simulink model "Simulation"  (R2016a)
settings: Solver=VariableStepAuto  StartTime=0.0  StopTime=5  FixedStep=1e-6  RelTol=1e-3
values from neighbouring files (symbols this model uses):
  B = 0    [Main.m]
  di_k_init = rand(2, 8)    [Main.m]
  G = (1/3)*[2 -1 -1; 0 sqrt(3) -sqrt(3)]    [Main.m]
  i_cmd_init = zeros(2, 3)    [Main.m]
  i_future_init = rand(2, 8)    [Main.m]
  i_k_init = rand(2, 8)    [Main.m]
  I_output = zeros(3, 1)    [Main.m]
  i_prev_init = rand(2, 1)    [Main.m]
  J = 0.0755    [Main.m]
  Ld = 0.04    [Main.m]
  Lq = 0.016    [Main.m]
  P = 3    [Main.m]
  R = 2.5    [Main.m]
  r_init = [0; 50; 0]    [Main.m]
  S_init = ones(3, 1)    [Main.m]
  Sensor_output = zeros(2, 1)    [Main.m]
  Ts = 100e-6    (= 0.0001)    [Main.m]
  V = 220    [Main.m]
libraries: simulink x1
settings Model: Creator=Raheel  LastModifiedBy=Raheel

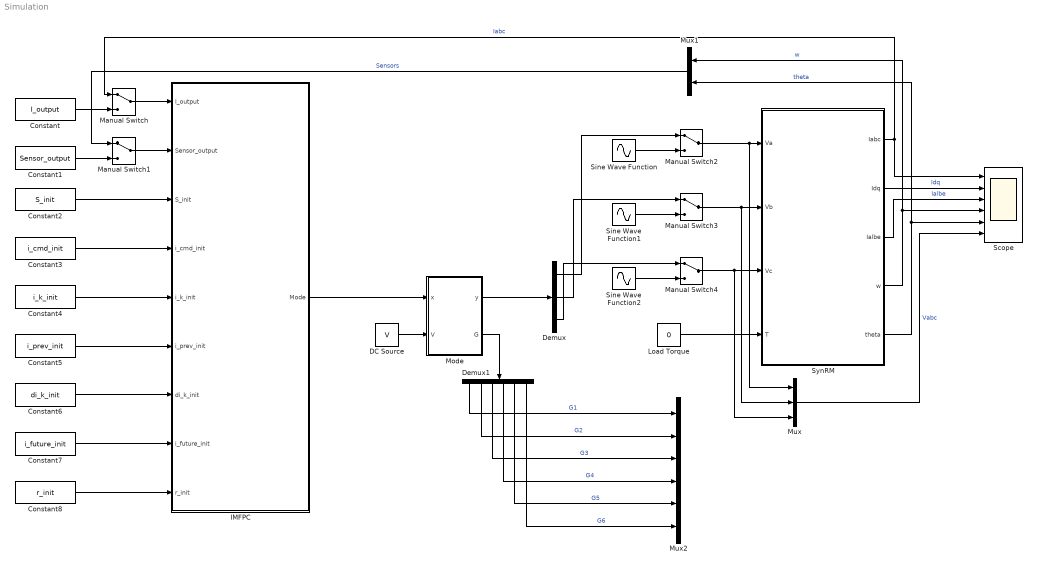
== system Simulation ==
  Constant : Constant  Value=I_output  VectorParams1D=off  SampleTime=Ts
  Constant1 : Constant  Value=Sensor_output  VectorParams1D=off  SampleTime=Ts
  Constant2 : Constant  Value=S_init  VectorParams1D=off  SampleTime=Ts
  Constant3 : Constant  Value=i_cmd_init  VectorParams1D=off  SampleTime=Ts
  Constant4 : Constant  Value=i_k_init  VectorParams1D=off  SampleTime=Ts
  Constant5 : Constant  Value=i_prev_init  SampleTime=Ts
  Constant6 : Constant  Value=di_k_init  SampleTime=Ts
  Constant7 : Constant  Value=i_future_init  SampleTime=Ts
  Constant8 : Constant  Value=r_init  SampleTime=Ts
  DC Source : Constant  Value=V  SampleTime=Ts
  Demux : Demux  Outputs=3
  Demux1 : Demux  Outputs=6
  IMFPC : Subsystem
  "Load Torque " : Constant  Value=0  SampleTime=0
  Manual Switch{,1..4} (5 alike) : ManualSwitch
  Mode : MATLAB Function  TreatAsAtomicUnit=on
  Mux : Mux  Inputs=3
  Mux1 : Mux  Inputs=2
  Mux2 : Mux  Inputs=6
  Scope : Scope  NumInputPorts=6
  Sine Wave Function : Sin  Amplitude=V  Frequency=50  SampleTime=0
  Sine Wave Function1 : Sin  Amplitude=V  Frequency=50  Phase=-2*pi/3  SampleTime=0
  Sine Wave Function2 : Sin  Amplitude=V  Frequency=50  Phase=2*pi/3  SampleTime=0
  SynRM : Subsystem
  wires:
  Constant8/1 -> IMFPC/9(r_init)
  Constant7/1 -> IMFPC/8(i_future_init)
  Constant6/1 -> IMFPC/7(di_k_init)
  Constant5/1 -> IMFPC/6(i_prev_init)
  Constant4/1 -> IMFPC/5(i_k_init)
  Constant3/1 -> IMFPC/4(i_cmd_init)
  Constant2/1 -> IMFPC/3(S_init)
  "Load Torque "/1 -> SynRM/4(T)
  Sine Wave Function1/1 -> Manual Switch3/2
  Sine Wave Function/1 -> Manual Switch2/2
  Sine Wave Function2/1 -> Manual Switch4/2
  SynRM/1(Iabc) -> Scope/1, Manual Switch/1  "Iabc"
  SynRM/4(w) -> Mux1/1, Scope/4  "w"
  SynRM/5(theta) -> Mux1/2, Scope/5  "theta"
  SynRM/3(Ialbe) -> Scope/3  "Ialbe"
  SynRM/2(Idq) -> Scope/2  "Idq"
  Mux/1 -> Scope/6  "Vabc"
  Constant/1 -> Manual Switch/2
  Manual Switch/1 -> IMFPC/1(I_output)
  Manual Switch1/1 -> IMFPC/2(Sensor_output)
  Constant1/1 -> Manual Switch1/2
  Manual Switch2/1 -> Mux/1, SynRM/1(Va)
  Manual Switch3/1 -> Mux/2, SynRM/2(Vb)
  Manual Switch4/1 -> Mux/3, SynRM/3(Vc)
  IMFPC/1(Mode) -> Mode/1(x)
  DC Source/1 -> Mode/2(V)
  Mode/1(y) -> Demux/1
  Demux/1 -> Manual Switch2/1
  Mux1/1 -> Manual Switch1/1  "Sensors"
  Demux/2 -> Manual Switch3/1
  Demux/3 -> Manual Switch4/1
  Mode/2(G) -> Demux1/1
  Demux1/6 -> Mux2/6  "G6"
  Demux1/5 -> Mux2/5  "G5"
  Demux1/4 -> Mux2/4  "G4"
  Demux1/3 -> Mux2/3  "G3"
  Demux1/2 -> Mux2/2  "G2"
  Demux1/1 -> Mux2/1  "G1"

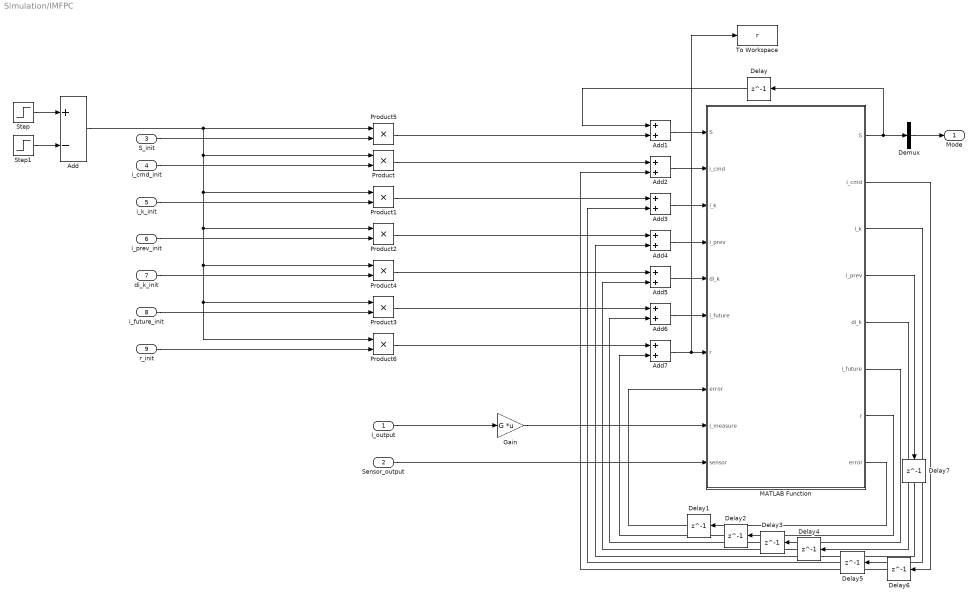
== system Simulation/IMFPC ==
  I_output : Inport
  Sensor_output : Inport  Port=2
  S_init : Inport  Port=3
  i_cmd_init : Inport  Port=4
  i_k_init : Inport  Port=5
  i_prev_init : Inport  Port=6
  di_k_init : Inport  Port=7
  i_future_init : Inport  Port=8
  r_init : Inport  Port=9
  Add : Sum  Inputs=+-
  Add{1..7} (7 alike) : Sum
  Delay{,1..7} (8 alike) : Delay  DelayLength=1  InitialCondition=0  SampleTime=Ts
  Demux : Demux  Outputs=3
  Gain : Gain  Gain=G  Multiplication=Matrix(K*u)
  MATLAB Function : MATLAB Function  TreatAsAtomicUnit=on
  Product{,1..6} (7 alike) : Product
  Step : Step  Time=0  SampleTime=Ts  ZeroCross=off
  Step1 : Step  Time=Ts  SampleTime=Ts  ZeroCross=off
  To Workspace : ToWorkspace  VariableName=r  SaveFormat=Timeseries  SampleTime=-1
  Mode : Outport
  wires:
  Step/1 -> Add/1
  Step1/1 -> Add/2
  MATLAB Function/8(error) -> Delay1/1
  MATLAB Function/1(S) -> Delay/1, Demux/1
  Add/1 -> Product1/1, Product6/1, Product3/1, Product4/1, Product2/1, Product/1, Product5/1
  Product5/1 -> Add1/2
  Add1/1 -> MATLAB Function/1("S ")
  Add2/1 -> MATLAB Function/2("i_cmd ")
  Add3/1 -> MATLAB Function/3("i_k ")
  Add4/1 -> MATLAB Function/4("i_prev ")
  Add5/1 -> MATLAB Function/5("di_k ")
  Add6/1 -> MATLAB Function/6("i_future ")
  Add7/1 -> To Workspace/1, MATLAB Function/7("r ")
  Product/1 -> Add2/1
  Product1/1 -> Add3/1
  Product2/1 -> Add4/1
  Product4/1 -> Add5/1
  Product3/1 -> Add6/1
  Product6/1 -> Add7/1
  MATLAB Function/2(i_cmd) -> Delay6/1
  MATLAB Function/3(i_k) -> Delay5/1
  MATLAB Function/5(di_k) -> Delay4/1
  MATLAB Function/6(i_future) -> Delay3/1
  MATLAB Function/7(r) -> Delay2/1
  Gain/1 -> MATLAB Function/9(i_measure)
  S_init/1 -> Product5/2
  i_cmd_init/1 -> Product/2
  r_init/1 -> Product6/2
  i_future_init/1 -> Product3/2
  di_k_init/1 -> Product4/2
  i_prev_init/1 -> Product2/2
  i_k_init/1 -> Product1/2
  Demux/2 -> Mode/1
  I_output/1 -> Gain/1
  Sensor_output/1 -> MATLAB Function/10(sensor)
  Delay/1 -> Add1/1
  Delay1/1 -> MATLAB Function/8("error ")
  Delay2/1 -> Add7/2
  Delay3/1 -> Add6/2
  Delay4/1 -> Add5/2
  Delay5/1 -> Add3/2
  Delay6/1 -> Add2/2
  MATLAB Function/4(i_prev) -> Delay7/1
  Delay7/1 -> Add4/2

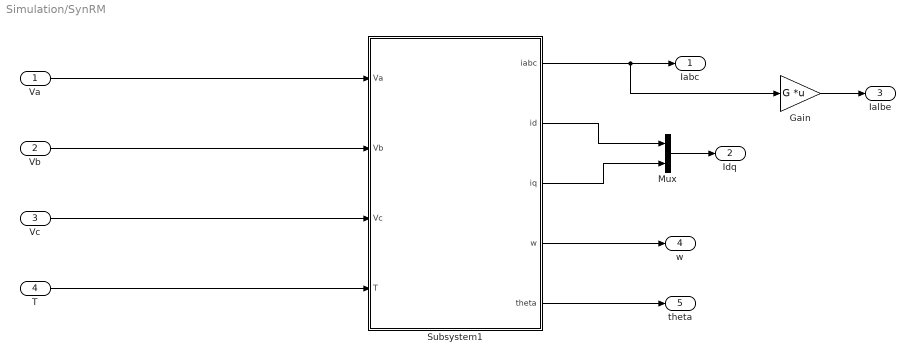
== system Simulation/SynRM ==
  Va : Inport
  Vb : Inport  Port=2
  Vc : Inport  Port=3
  T : Inport  Port=4
  Gain : Gain  Gain=G  Multiplication=Matrix(K*u)
  Mux : Mux  Inputs=2
  Subsystem1 : Subsystem
  Iabc : Outport
  Idq : Outport  Port=2
  Ialbe : Outport  Port=3
  w : Outport  Port=4
  theta : Outport  Port=5
  wires:
  Va/1 -> Subsystem1/1(Va)
  Vb/1 -> Subsystem1/2(Vb)
  Vc/1 -> Subsystem1/3(Vc)
  T/1 -> Subsystem1/4(T)
  Subsystem1/1(iabc) -> Gain/1, Iabc/1
  Subsystem1/2(id) -> Mux/1
  Subsystem1/3(iq) -> Mux/2
  Mux/1 -> Idq/1
  Gain/1 -> Ialbe/1
  Subsystem1/5(theta) -> theta/1
  Subsystem1/4(w) -> w/1

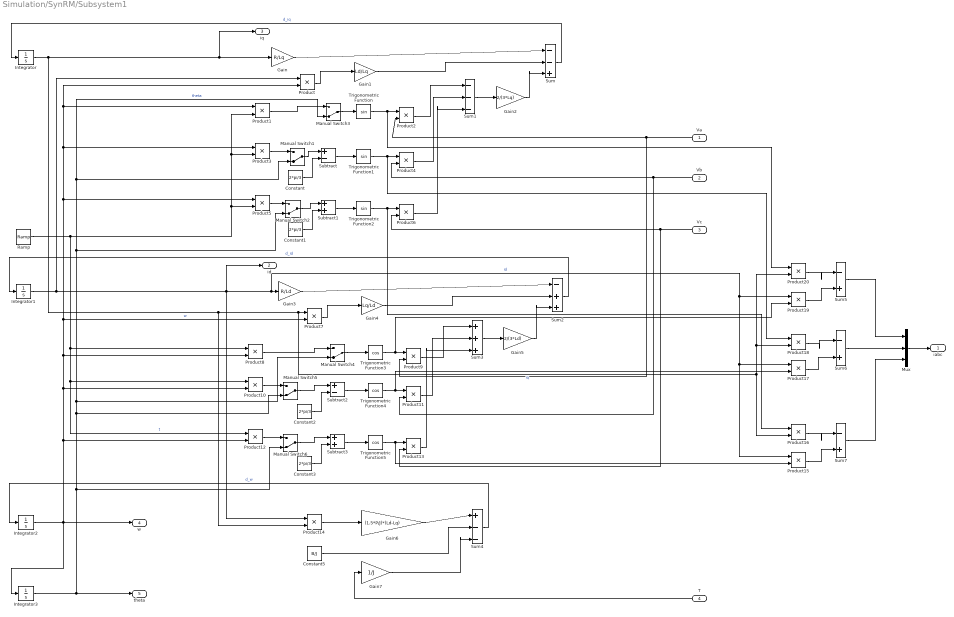
== system Simulation/SynRM/Subsystem1 ==
  Va : Inport
  Vb : Inport  Port=2
  Vc : Inport  Port=3
  T : Inport  Port=4
  Constant{,1..3} (4 alike) : Constant  Value=2*pi/3  SampleTime=0
  Constant5 : Constant  Value=B/J  SampleTime=0
  Gain : Gain  Gain=R/Lq
  Gain1 : Gain  Gain=Ld/Lq
  Gain2 : Gain  Gain=2/(3*Lq)
  Gain3 : Gain  Gain=R/Ld
  Gain4 : Gain  Gain=Lq/Ld
  Gain5 : Gain  Gain=2/(3*Ld)
  Gain6 : Gain  Gain=(1.5*P/J)*(Ld-Lq)
  Gain7 : Gain  Gain=1/J
  Integrator{,1..3} (4 alike) : Integrator
  Manual Switch{1..6} (6 alike) : ManualSwitch  CurrentSetting=0
  Mux : Mux  Inputs=3
  Product{,1..20} (21 alike) : Product
  Ramp : simulink/Sources/Ramp  slope=1  start=0  X0=0
  Subtract : Sum  Inputs=+-
  Subtract1 : Sum
  Subtract2 : Sum  Inputs=+-
  Subtract3 : Sum
  Sum : Sum  Inputs=|--+
  Sum1 : Sum  Inputs=|---
  Sum2 : Sum  Inputs=|-++
  Sum3 : Sum  Inputs=|+++
  Sum4 : Sum  Inputs=|+--
  Sum5 : Sum  Inputs=|-+
  Sum6 : Sum  Inputs=|-+
  Sum7 : Sum  Inputs=|-+
  Trigonometric Function : Trigonometry
  Trigonometric Function1 : Trigonometry
  Trigonometric Function2 : Trigonometry
  Trigonometric Function3 : Trigonometry  Operator=cos
  Trigonometric Function4 : Trigonometry  Operator=cos
  Trigonometric Function5 : Trigonometry  Operator=cos
  iabc : Outport
  id : Outport  Port=2
  iq : Outport  Port=3
  w : Outport  Port=4
  theta : Outport  Port=5
  wires:
  Integrator/1 -> Product14/2, Product16/2, Product20/2, Product18/2, Product7/1, iq/1, Gain/1  "iq"
  Gain/1 -> Sum/1
  Gain1/1 -> Sum/2
  Product/1 -> Gain1/1
  Ramp/1 -> Product8/1, Product10/1, Product12/1, Product1/2, Product3/2, Product5/2  "t"
  Constant/1 -> Subtract/2
  Trigonometric Function1/1 -> Product18/1, Product4/1
  Constant1/1 -> Subtract1/2
  Trigonometric Function2/1 -> Product16/1, Product6/1
  Product2/1 -> Sum1/1
  Product4/1 -> Sum1/2
  Product6/1 -> Sum1/3
  Sum1/1 -> Gain2/1
  Gain2/1 -> Sum/3
  Sum/1 -> Integrator/1  "d_iq"
  Integrator1/1 -> Product14/1, Product19/1, Product17/1, Product15/1, Gain3/1, id/1, Product/1  "id"
  Gain3/1 -> Sum2/1
  Gain4/1 -> Sum2/2
  Product7/1 -> Gain4/1
  Integrator2/1 -> w/1, Integrator3/1, Product10/2, Product8/2, Product7/2, Product5/1, Product3/1, Product1/1, Product/2, Product12/2  "w"
  Trigonometric Function3/1 -> Product19/2, Product9/1
  Va/1 -> Product9/2, Product2/2
  Constant2/1 -> Subtract2/2
  Trigonometric Function4/1 -> Product17/2, Product11/1
  Vb/1 -> Product11/2, Product4/2
  Constant3/1 -> Subtract3/2
  Trigonometric Function5/1 -> Product15/2, Product13/1
  Vc/1 -> Product13/2, Product6/2
  Product9/1 -> Sum3/1
  Product11/1 -> Sum3/2
  Product13/1 -> Sum3/3
  Sum3/1 -> Gain5/1
  Gain5/1 -> Sum2/3
  Sum2/1 -> Integrator1/1  "d_id"
  Product14/1 -> Gain6/1
  Gain6/1 -> Sum4/1
  Sum4/1 -> Integrator2/1  "d_w"
  Constant5/1 -> Sum4/2
  Gain7/1 -> Sum4/3
  T/1 -> Gain7/1
  Integrator3/1 -> Manual Switch6/2, Manual Switch5/2, Manual Switch4/2, Manual Switch2/2, Manual Switch1/2, Manual Switch3/2, theta/1  "theta"
  Trigonometric Function/1 -> Product20/1, Product2/1
  Product20/1 -> Sum5/1
  Product19/1 -> Sum5/2
  Product18/1 -> Sum6/1
  Product17/1 -> Sum6/2
  Product16/1 -> Sum7/1
  Product15/1 -> Sum7/2
  Sum5/1 -> Mux/1
  Mux/1 -> iabc/1
  Sum6/1 -> Mux/2
  Sum7/1 -> Mux/3
  Manual Switch3/1 -> Trigonometric Function/1
  Product1/1 -> Manual Switch3/1
  Manual Switch4/1 -> Trigonometric Function3/1
  Product8/1 -> Manual Switch4/1
  Product3/1 -> Manual Switch1/1
  Manual Switch1/1 -> Subtract/1
  Subtract/1 -> Trigonometric Function1/1
  Product5/1 -> Manual Switch2/1
  Subtract1/1 -> Trigonometric Function2/1
  Manual Switch2/1 -> Subtract1/1
  Product10/1 -> Manual Switch5/1
  Subtract2/1 -> Trigonometric Function4/1
  Manual Switch5/1 -> Subtract2/1
  Product12/1 -> Manual Switch6/1
  Subtract3/1 -> Trigonometric Function5/1
  Manual Switch6/1 -> Subtract3/1

== matlab function Simulation/Mode ==
  data: x input; y output; V input; G output
function [y, G]=Mode(x, V)

switch x
    case 1
        y=[0; 0; 0];
        G=[0; 1; 0; 1; 0; 1];
    case 2
        y=[2*V/3; -V/3; -V/3];
        G=[1; 0; 0; 1; 0; 1];
    case 3
        y=[-2*V/3; V/3; V/3];
        G=[0; 1; 1; 0; 1; 0];
    case 4
        y=[-V/3; 2*V/3; -V/3];
        G=[0; 1; 1; 0; 0; 1];
    case 5
        y=[V/3; -2*V/3; V/3];
        G=[1; 0; 0; 1; 1; 0];
    case 6
        y=[-V/3; -V/3; 2*V/3];
        G=[0; 1; 0; 1; 1; 0];
    case 7
        y=[V/3; V/3; -2*V/3];
        G=[1; 0; 1; 0; 0; 1];
    case 8
        y=[0; 0; 0];
        G=[1; 0; 1; 0; 1; 0];
    otherwise
        disp('Error! Incorrect mode inserted');
        y=[0; 0; 0];
        G=[1; 0; 1; 0; 1; 0];
end

end

== matlab function Simulation/IMFPC/MATLAB Function ==
  data: S input; S output; i_cmd input; i_k input; i_prev input; di_k input; i_future input; r input; error input; i_measure input; sensor input; i_cmd output; i_k output; i_prev output; di_k output; i_future output; r output; error output
%% Details about the algorithm IMPFC
% 1) S is a vector. S(1)=Present mode, S(2)=Mode to be applied, S(3)=Mode calculated
% 2) i_cmd is a matrix. i_cmd(a, 1)=i*(k), i_cmd(a, 2)=i*(k-1), i_cmd(a, 3)=i*(k-2)
%    a=1 means alpha, a=2 means beta.
% 3) i_k is a matrix. i_k(a, b) are the predicted values at present instant.
%    a=1 means alpha, a=2 means beta, b represents the conducting mode.
% 4) i_measure is a vector. i_measure(a) is the current measurement sample.
%    a=1 means alpha, a=2 means beta.
% 5) i_prev is a vector. i_prev(a) is the previous measurement sample.
%    a=1 means alpha, a=2 means beta.
% 6) di_prev is a matrix. di_prev(a, b) is the current variation for previous time instant.
%    a=1 means alpha, a=2 means beta.
% 7) i_future is a matrix. i_future(a, b) are the predicted values at next instant.
%    a=1 means alpha, a=2 means beta, b represents the conducting mode.
% 8) r is a vector. r(1) takes on values from 0 to r(2). r(2)=50. 

function [S, i_cmd, i_k, i_prev, di_k, i_future, r, error]=IMFPC(S, i_cmd, i_k, i_prev, di_k, i_future, r, error, i_measure, sensor)
r(3)=r(3)+1;

if r(3)<=20000
    wref=25;
else
    wref=50;
end
%% Parameters
idref=5;
Kp=0;
Ki=0.5;

%% Read stator current
S(1)=S(2);
i_k(:, S(1))=i_measure;
temp=i_future;

%% Current command calculations
if r(3)==1
    error0=0;
else
    error0=error;
end
offset=0;
w=sensor(1);
theta=sensor(2);
error=wref-w+offset;
iqref=error*Kp+(error+error0)*Ki;
ialbe_ref=DQ2Clark(theta, idref, iqref);
i_cmd(:, 1)=ialbe_ref;

%% Apply conduction mode
S(2)=S(3);

%% Compute and update current variations
di_prev=di_k;
di_k(:, S(1))=i_k(:, S(1))-i_prev;
    
%% Generate the current command
i_cmd_k=6*i_cmd(:, 1)-8*i_cmd(:, 2)+3*i_cmd(:, 3);

%% Reset g_old and future stator current prediction
g=zeros(1, 8);
for j=1:8
    i_future(:, j)=i_k(:, S(1))+di_k(:, S(2))+di_k(:, j);
    g(j)=sum(abs(i_cmd_k-i_future(:, j)));
end
[gmin, S(3)]=min(g);

%% Checking stagnant current mode  
r(1)=r(1)+1;
if r(1)==r(2)
    for l=1:8
        if di_prev(1, l)==di_k(1, l) && di_prev(2, l)==di_k(2, l)
                S(3)=l;
        end
    end
    r(1)=0;
end

%% Updation of variables
i_cmd(:, 3)=i_cmd(:, 2);
i_cmd(:, 2)=i_cmd(:, 1);
i_prev=i_k(:, S(1));
i_k=temp;

end
